simulink model "project_1_part5"  (R2021b)
settings: Solver=ode3  StartTime=0.0  StopTime=10.0  FixedStep=0.01  RelTol=1e-3
undefined symbols (not defined in the file or in its folder): DiscIntNeverNeededParam
libraries: simulink x1
settings Model: Creator=jlkbo  LastModifiedBy=jlkbo

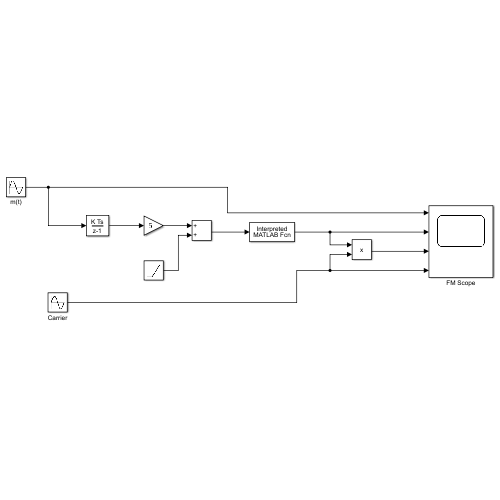
[thumbnail: Simulink's stored preview of the top-level diagram]
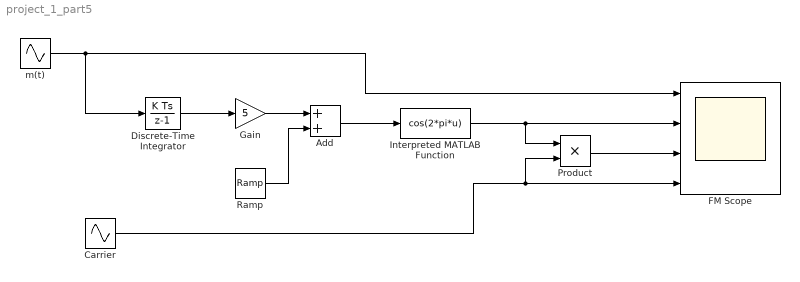
== system project_1_part5 ==
  Add : Sum
  Carrier : Sin  Frequency=25  SampleTime=0
  Discrete-Time Integrator : DiscreteIntegrator  SampleTime=-1  ICPrevOutput=DiscIntNeverNeededParam  ICPrevScaledInput=DiscIntNeverNeededParam
  FM Scope : Scope  NumInputPorts=4
  Gain : Gain  Gain=5
  Interpreted MATLAB Function : MATLABFcn  MATLABFcn=cos(2*pi*u)
  Product : Product
  Ramp : simulink/Sources/Ramp  slope=10  start=0  InitialOutput=0
  m(t) : Sin  Amplitude=2  Frequency=2*pi  SampleTime=0
  wires:
  Gain/1 -> Add/1
  m(t)/1 -> Discrete-Time Integrator/1, FM Scope/1
  Carrier/1 -> Product/2, FM Scope/4
  Discrete-Time Integrator/1 -> Gain/1
  Ramp/1 -> Add/2
  Add/1 -> Interpreted MATLAB Function/1
  Interpreted MATLAB Function/1 -> Product/1, FM Scope/2
  Product/1 -> FM Scope/3
